simulink model "LeftTurnScenario_withMultipleObjects"  (R2020b)
settings: Solver=FixedStepDiscrete  StartTime=0.0  StopTime=10.0  RelTol=1e-3
model workspace (MAT data in the model file):
  firstWarning = 1
  originalScenarioChecksum = 'AA0118080BFCF80951182C28590E18E5'
undefined symbols (not defined in the file or in its folder): driving
libraries: drivingscenarioandsensors x9
(part 1 of 3)
settings Model: Creator=ragha  LastModifiedBy=ragha

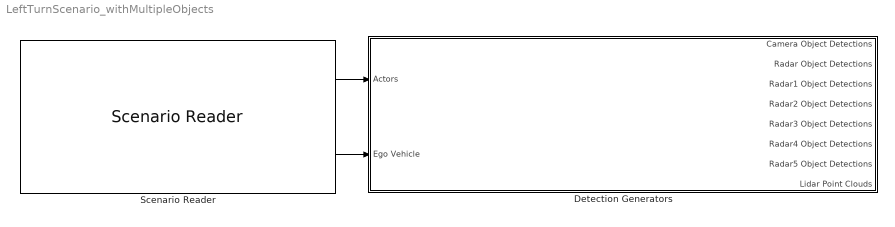
== system LeftTurnScenario_withMultipleObjects ==
  Detection Generators : Subsystem
  Scenario Reader : drivingscenarioandsensors/Scenario Reader  ScenarioSource=From file  ScenarioFileName=A:\desktop\Dorle controls\Simulink lidar test\YESSSS\Egomap\OCT1st\Success Test from createegocentricocc_matlabfile_Oct4th\LeftTurnScenarioTrial11.mat  ScenarioVariableName=scenario  OutputCoordinateSystem=Vehicle coordinates  EgoVehicleSource=Scenario  EgoVehicleActorID=1  OrientVehiclesOnRoad=off  OutputEgoVehiclePose=on  SampleTime=0.1  LaneBoundaryOutput=None  LaneBoundaryDistance=0:0.5:9.5  LaneBoundaryLocation=Center of lane markings  BusNameSource=Auto  BusName=BusActors  BusName2Source=Auto  BusName2=BusLaneBoundaries  BusName3Source=Auto  BusName3=BusEgoActor  ShowCoordinateLabels=on  SimulateUsing=Interpreted execution
  wires:
  Scenario Reader/1 -> Detection Generators/1(Actors)
  Scenario Reader/2 -> Detection Generators/2(Ego Vehicle)
